simulink model "Elevator_correction"  (R2024b)
settings: Solver=VariableStepAuto  StartTime=0.0  StopTime=SIM.Tmax  MaxStep=SIM.Step_max  RelTol=1e-3
InitFcn:
  | Initialisation
values from neighbouring files (symbols this model uses):
  Kr = 12    [Initialisation.m]
  Mc = 1000.0    (= 1000)    [Initialisation.m]
  Me = 800.0    (= 800)    [Initialisation.m]
  Rp = 0.1    [Initialisation.m]
  Ured = 3.0/pi*sqrt(2.0)*sqrt(3.0)*230.0    [Initialisation.m]
undefined symbols (not defined in the file or in its folder): cycle, IN_filter, MOT, Scap
settings Model: Creator=philippe.barrade  LastModifiedBy=philippe.barrade
settings SolverCC: AlgebraicLoopSolver=TrustRegion
settings DataIOCC: ReturnWorkspaceOutputs=off
settings DebuggingCC: UnconnectedInputMsg=warning  UnconnectedOutputMsg=warning  UnconnectedLineMsg=warning  ArithmeticOperatorsInVariantConditions=warning
settings ModelReferenceCC: EnableRefExpFcnMdlSchedulingChecks=on
settings SFSimCC: SimUseLocalCustomCode=off  CustomCodeUndefinedFunction=UseInterfaceOnly
settings RTWCC: RTWUseLocalCustomCode=off  GPUComputeCapability=3.5
settings CodeAppCC: StateflowObjectComments=on

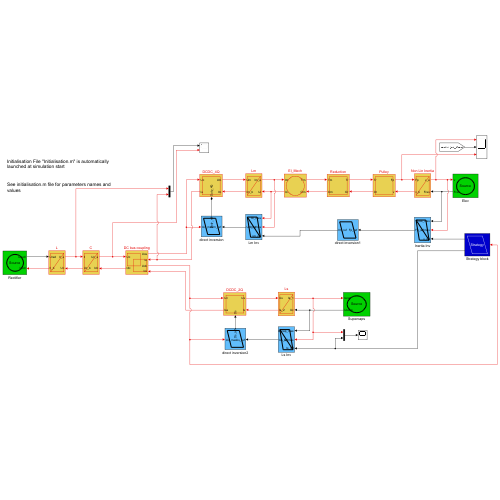
[thumbnail: Simulink's stored preview of the top-level diagram]
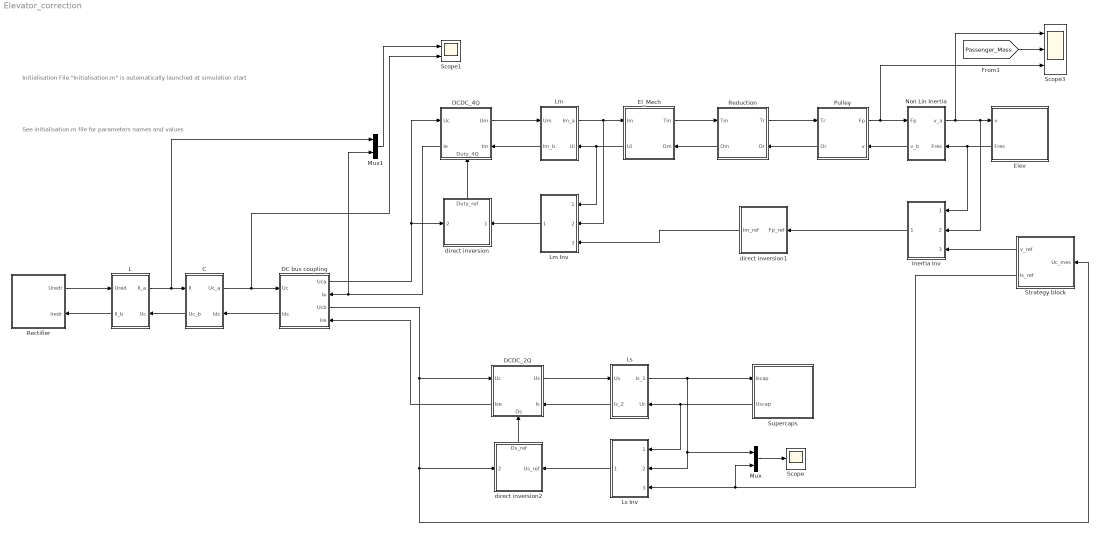
== system Elevator_correction ==
  note: Initialisation File "Initialisation.m" is automatically launched at simulation start
  note: See initialisation.m file for parameters names and values
  C : Subsystem  mask(CM){}
      settings: PortSchema="{\"entries\":[{\"content\":{\"sides\":[{\"content\":{\"connectorIds\":[\"In1\",\"Out2\"]},\"type\":\"ConnectorPlacement.EquallySpacedRectSide\",\"uuid\":\"af5f45e0-9d2b-440a-ad04-5e1193860bd0\"},{\"content\":{\"connectorIds\":[\"Out1\",\"In2\"],\"side\":\"RIGHT\"},\"type\":\"ConnectorPlacement.EquallySpacedRectSide\",\"uuid\":\"8de6af24-0ac6-4b19-a2ba-5daa5911acc7\"},{\"content\":{\"connectorIds\":[],\"side\":\"TOP\"},\"type\":\"ConnectorPlacement.EquallySpacedRectSide\",\"uuid\":\"acb7e0d5-07ac-49d2-a96a-2a7cab5175a2\"}]},\"type\":\"ConnectorPlacement.EquallySpacedConnector\",\"uuid\":\"c84922a6-ff22-4e39-b94d-9f3f8f0085b4\"}],\"packageUris\":[\"http://schema.mathworks.com/mf0/Connector/R2020b\"],\"version\":\"1.0\"}"
      mask Display: plot(0,0,100,100,[10,10,90,90,10],[90,10,10,90,90], [10,90],[10,90])
  DC bus coupling : Subsystem  mask(CM){}
      settings: PortSchema="{\"entries\":[{\"content\":{\"sides\":[{\"content\":{\"connectorIds\":[\"In1\",\"Out3\"]},\"type\":\"ConnectorPlacement.EquallySpacedRectSide\",\"uuid\":\"a0cc6eb3-0f35-4a31-afc0-a3cae9b9d5bb\"},{\"content\":{\"connectorIds\":[\"Out1\",\"In2\",\"Out2\",\"In3\"],\"side\":\"RIGHT\"},\"type\":\"ConnectorPlacement.EquallySpacedRectSide\",\"uuid\":\"f0fc86c1-6f18-402b-9eea-d081ace87e62\"},{\"content\":{\"connectorIds\":[],\"side\":\"TOP\"},\"type\":\"ConnectorPlacement.EquallySpacedRectSide\",\"uuid\":\"dfd8824c-ea43-4486-a7b0-05621e67d875\"}]},\"type\":\"ConnectorPlacement.EquallySpacedConnector\",\"uuid\":\"18c849d2-2a12-4239-b86e-b7a06eec8617\"}],\"packageUris\":[\"http://schema.mathworks.com/mf0/Connector/R2020b\"],\"version\":\"1.0\"}"
      mask Display: plot(0,0,100,100,[35,35,95,95,35],[65,10,10,65,65], [5,5,65,65,5],[90,35,35,90,90])
  DCDC_2Q : Subsystem  mask(Hacheur){}
      settings: PortSchema="{\"entries\":[{\"content\":{\"sides\":[{\"content\":{\"connectorIds\":[\"In1\",\"Out2\"]},\"type\":\"ConnectorPlacement.EquallySpacedRectSide\",\"uuid\":\"18b8dea3-c73c-4489-bf41-881ff948b4bd\"},{\"content\":{\"connectorIds\":[\"Out1\",\"In3\"],\"side\":\"RIGHT\"},\"type\":\"ConnectorPlacement.EquallySpacedRectSide\",\"uuid\":\"3421d2ab-808d-44dd-9f9d-6c595338ccbb\"},{\"content\":{\"connectorIds\":[],\"side\":\"TOP\"},\"type\":\"ConnectorPlacement.EquallySpacedRectSide\",\"uuid\":\"948f89bd-2b52-44e4-9785-94aa615b18dd\"},{\"content\":{\"connectorIds\":[\"In2\"],\"side\":\"BOTTOM\"},\"type\":\"ConnectorPlacement.EquallySpacedRectSide\",\"uuid\":\"f632fc7f-d418-4a7f-b063-8935e3a44c68\"}]},\"type\":\"ConnectorPlacement.EquallySpacedConnector\",\"uuid\":\"698b37cd-a833-4d3c-8172-8b0b4e01ebf3\"}],\"packageUris\":[\"http://schema.mathworks.com/mf0/Connector/R2020b\"],\"version\":\"1.0\"}"
      mask Display: plot(0,0,100,100,[10,10,90,90,10],[90,10,10,90,90])
  DCDC_4Q : Subsystem  mask(Hacheur){}
      settings: PortSchema="{\"entries\":[{\"content\":{\"sides\":[{\"content\":{\"connectorIds\":[\"In1\",\"Out2\"]},\"type\":\"ConnectorPlacement.EquallySpacedRectSide\",\"uuid\":\"18b8dea3-c73c-4489-bf41-881ff948b4bd\"},{\"content\":{\"connectorIds\":[\"Out1\",\"In3\"],\"side\":\"RIGHT\"},\"type\":\"ConnectorPlacement.EquallySpacedRectSide\",\"uuid\":\"3421d2ab-808d-44dd-9f9d-6c595338ccbb\"},{\"content\":{\"connectorIds\":[],\"side\":\"TOP\"},\"type\":\"ConnectorPlacement.EquallySpacedRectSide\",\"uuid\":\"948f89bd-2b52-44e4-9785-94aa615b18dd\"},{\"content\":{\"connectorIds\":[\"In2\"],\"side\":\"BOTTOM\"},\"type\":\"ConnectorPlacement.EquallySpacedRectSide\",\"uuid\":\"2b91a71a-e743-46c5-9fd2-ea2ea7735bb5\"}]},\"type\":\"ConnectorPlacement.EquallySpacedConnector\",\"uuid\":\"698b37cd-a833-4d3c-8172-8b0b4e01ebf3\"}],\"packageUris\":[\"http://schema.mathworks.com/mf0/Connector/R2020b\"],\"version\":\"1.0\"}"
      mask Display: plot(0,0,100,100,[10,10,90,90,10],[90,10,10,90,90])
  El_Mech : Subsystem
      settings: PortSchema="{\"entries\":[{\"content\":{\"sides\":[{\"content\":{\"connectorIds\":[\"In1\",\"Out2\"]},\"type\":\"ConnectorPlacement.EquallySpacedRectSide\",\"uuid\":\"af5f45e0-9d2b-440a-ad04-5e1193860bd0\"},{\"content\":{\"connectorIds\":[\"Out1\",\"In2\"],\"side\":\"RIGHT\"},\"type\":\"ConnectorPlacement.EquallySpacedRectSide\",\"uuid\":\"8de6af24-0ac6-4b19-a2ba-5daa5911acc7\"},{\"content\":{\"connectorIds\":[],\"side\":\"TOP\"},\"type\":\"ConnectorPlacement.EquallySpacedRectSide\",\"uuid\":\"acb7e0d5-07ac-49d2-a96a-2a7cab5175a2\"}]},\"type\":\"ConnectorPlacement.EquallySpacedConnector\",\"uuid\":\"c84922a6-ff22-4e39-b94d-9f3f8f0085b4\"}],\"packageUris\":[\"http://schema.mathworks.com/mf0/Connector/R2020b\"],\"version\":\"1.0\"}"
      mask Display: plot(0,0,100,100, 1.4*[50,57.68,60.77,63.08,64.97,66.58,68,69.26,70.4, 	71.42,72.36,78.28,80,78.28,72.36,71.42,70.4, 	69.26,68,66.58,64.97,63.08,60.77,57.68,50,42.32, 	39.23,36.92,35.03,33.42,32,30.74,29.6,28.58, 	27.64,21.72,20,21.72,27.64,28.58,29.6,30.74,32, 	33.42,35.03,36.92,39.23,42.32,50]-20, 1.4*[20,21,22,23,24,25,26,27,28,29,30,40,50,60,70,71,72, 	73,74,75,76,77,78,79,80,79,78,77,76,75,74,73,72, 	71,70,60,50,40,30,29,28,27,26,25,24,23,22,21,20]-20)
  Elev : Subsystem
      settings: PortSchema="{\"entries\":[{\"content\":{\"sides\":[{\"content\":{\"connectorIds\":[\"In1\",\"Out1\"]},\"type\":\"ConnectorPlacement.EquallySpacedRectSide\",\"uuid\":\"5a8fdec0-a98b-43d7-a4cd-372895ae0c1b\"},{\"content\":{\"connectorIds\":[],\"side\":\"RIGHT\"},\"type\":\"ConnectorPlacement.EquallySpacedRectSide\",\"uuid\":\"94211a24-953d-4ef9-bbc7-a0604a4babfb\"},{\"content\":{\"connectorIds\":[],\"side\":\"TOP\"},\"type\":\"ConnectorPlacement.EquallySpacedRectSide\",\"uuid\":\"df264a2a-7001-4aa8-9401-af00637c2dcd\"}]},\"type\":\"ConnectorPlacement.EquallySpacedConnector\",\"uuid\":\"5b044fdd-039d-40b1-9820-1583afc6fd22\"}],\"packageUris\":[\"http://schema.mathworks.com/mf0/Connector/R2020b\"],\"version\":\"1.0\"}"
      mask Display:
      | plot(0,0,100,100, 1.2*[50,57.68,60.77,63.08,64.97,66.58,68,69.26,70.4, 	71.42,72.36,78.28,80,78.28,72.36,71.42,70.4, 	69.26,68,66.58,64.97,63.08,60.77,57.68,50,42.32, 	39.23,36.92,35.03,33.42,32,30.74,29.6,28.58, 	27.64,21.72,20,21.72,27.64,28.58,29.6,30.74,32, 	33.42,35.03,36.92,39.23,42.32,50]-10, 1.2*[20,21,22,23,24,25,26,27,28,29,30,40,50,60,70,71,72, 	73,74,75,76,77,78,79,80,79,78,77,76,75,74,73,72, 	71,70,60,50,40,30,29,28,27,26,25,24,23,22,21,20]-10)
      | disp('Source')
  Inertia Inv : Subsystem
      mask Display: plot(0,0,100,100, [10,30,90,70,10,90],[90,10,10,90,90,10])
  L : Subsystem  mask(CM){}
      settings: PortSchema="{\"entries\":[{\"content\":{\"sides\":[{\"content\":{\"connectorIds\":[\"In1\",\"Out2\"]},\"type\":\"ConnectorPlacement.EquallySpacedRectSide\",\"uuid\":\"af5f45e0-9d2b-440a-ad04-5e1193860bd0\"},{\"content\":{\"connectorIds\":[\"Out1\",\"In2\"],\"side\":\"RIGHT\"},\"type\":\"ConnectorPlacement.EquallySpacedRectSide\",\"uuid\":\"8de6af24-0ac6-4b19-a2ba-5daa5911acc7\"},{\"content\":{\"connectorIds\":[],\"side\":\"TOP\"},\"type\":\"ConnectorPlacement.EquallySpacedRectSide\",\"uuid\":\"acb7e0d5-07ac-49d2-a96a-2a7cab5175a2\"}]},\"type\":\"ConnectorPlacement.EquallySpacedConnector\",\"uuid\":\"c84922a6-ff22-4e39-b94d-9f3f8f0085b4\"}],\"packageUris\":[\"http://schema.mathworks.com/mf0/Connector/R2020b\"],\"version\":\"1.0\"}"
      mask Display: plot(0,0,100,100,[10,10,90,90,10],[90,10,10,90,90], [10,90],[10,90])
  Lm : Subsystem  mask(CM){}
      settings: PortSchema="{\"entries\":[{\"content\":{\"sides\":[{\"content\":{\"connectorIds\":[\"In1\",\"Out2\"]},\"type\":\"ConnectorPlacement.EquallySpacedRectSide\",\"uuid\":\"af5f45e0-9d2b-440a-ad04-5e1193860bd0\"},{\"content\":{\"connectorIds\":[\"Out1\",\"In2\"],\"side\":\"RIGHT\"},\"type\":\"ConnectorPlacement.EquallySpacedRectSide\",\"uuid\":\"8de6af24-0ac6-4b19-a2ba-5daa5911acc7\"},{\"content\":{\"connectorIds\":[],\"side\":\"TOP\"},\"type\":\"ConnectorPlacement.EquallySpacedRectSide\",\"uuid\":\"acb7e0d5-07ac-49d2-a96a-2a7cab5175a2\"}]},\"type\":\"ConnectorPlacement.EquallySpacedConnector\",\"uuid\":\"c84922a6-ff22-4e39-b94d-9f3f8f0085b4\"}],\"packageUris\":[\"http://schema.mathworks.com/mf0/Connector/R2020b\"],\"version\":\"1.0\"}"
      mask Display: plot(0,0,100,100,[10,10,90,90,10],[90,10,10,90,90], [10,90],[10,90])
  Lm Inv : Subsystem
      mask Display: plot(0,0,100,100, [10,30,90,70,10,90],[90,10,10,90,90,10])
  Ls : Subsystem  mask(CM){}
      settings: PortSchema="{\"entries\":[{\"content\":{\"sides\":[{\"content\":{\"connectorIds\":[\"In1\",\"Out2\"]},\"type\":\"ConnectorPlacement.EquallySpacedRectSide\",\"uuid\":\"af5f45e0-9d2b-440a-ad04-5e1193860bd0\"},{\"content\":{\"connectorIds\":[\"Out1\",\"In2\"],\"side\":\"RIGHT\"},\"type\":\"ConnectorPlacement.EquallySpacedRectSide\",\"uuid\":\"8de6af24-0ac6-4b19-a2ba-5daa5911acc7\"},{\"content\":{\"connectorIds\":[],\"side\":\"TOP\"},\"type\":\"ConnectorPlacement.EquallySpacedRectSide\",\"uuid\":\"acb7e0d5-07ac-49d2-a96a-2a7cab5175a2\"}]},\"type\":\"ConnectorPlacement.EquallySpacedConnector\",\"uuid\":\"c84922a6-ff22-4e39-b94d-9f3f8f0085b4\"}],\"packageUris\":[\"http://schema.mathworks.com/mf0/Connector/R2020b\"],\"version\":\"1.0\"}"
      mask Display: plot(0,0,100,100,[10,10,90,90,10],[90,10,10,90,90], [10,90],[10,90])
  Ls Inv : Subsystem
      mask Display: plot(0,0,100,100, [10,30,90,70,10,90],[90,10,10,90,90,10])
  Mux : Mux  Inputs=2
  Mux1 : Mux  Inputs=2
  Non Lin Inertia : Subsystem  mask(CM){}
      settings: PortSchema="{\"entries\":[{\"content\":{\"sides\":[{\"content\":{\"connectorIds\":[\"In1\",\"Out2\"]},\"type\":\"ConnectorPlacement.EquallySpacedRectSide\",\"uuid\":\"af5f45e0-9d2b-440a-ad04-5e1193860bd0\"},{\"content\":{\"connectorIds\":[\"Out1\",\"In2\"],\"side\":\"RIGHT\"},\"type\":\"ConnectorPlacement.EquallySpacedRectSide\",\"uuid\":\"8de6af24-0ac6-4b19-a2ba-5daa5911acc7\"},{\"content\":{\"connectorIds\":[],\"side\":\"TOP\"},\"type\":\"ConnectorPlacement.EquallySpacedRectSide\",\"uuid\":\"acb7e0d5-07ac-49d2-a96a-2a7cab5175a2\"}]},\"type\":\"ConnectorPlacement.EquallySpacedConnector\",\"uuid\":\"c84922a6-ff22-4e39-b94d-9f3f8f0085b4\"}],\"packageUris\":[\"http://schema.mathworks.com/mf0/Connector/R2020b\"],\"version\":\"1.0\"}"
      mask Display: plot(0,0,100,100,[10,10,90,90,10],[90,10,10,90,90], [10,90],[10,90])
  Pulley : Subsystem  mask(Hacheur){}
      settings: PortSchema="{\"entries\":[{\"content\":{\"sides\":[{\"content\":{\"connectorIds\":[\"In1\",\"Out2\"]},\"type\":\"ConnectorPlacement.EquallySpacedRectSide\",\"uuid\":\"af5f45e0-9d2b-440a-ad04-5e1193860bd0\"},{\"content\":{\"connectorIds\":[\"Out1\",\"In2\"],\"side\":\"RIGHT\"},\"type\":\"ConnectorPlacement.EquallySpacedRectSide\",\"uuid\":\"8de6af24-0ac6-4b19-a2ba-5daa5911acc7\"},{\"content\":{\"connectorIds\":[],\"side\":\"TOP\"},\"type\":\"ConnectorPlacement.EquallySpacedRectSide\",\"uuid\":\"acb7e0d5-07ac-49d2-a96a-2a7cab5175a2\"}]},\"type\":\"ConnectorPlacement.EquallySpacedConnector\",\"uuid\":\"c84922a6-ff22-4e39-b94d-9f3f8f0085b4\"}],\"packageUris\":[\"http://schema.mathworks.com/mf0/Connector/R2020b\"],\"version\":\"1.0\"}"
      mask Display: plot(0,0,100,100,[10,10,90,90,10],[90,10,10,90,90])
  Rectifier : Subsystem
      settings: PortSchema="{\"entries\":[{\"content\":{\"sides\":[{\"content\":{\"connectorIds\":[]},\"type\":\"ConnectorPlacement.EquallySpacedRectSide\",\"uuid\":\"5a8fdec0-a98b-43d7-a4cd-372895ae0c1b\"},{\"content\":{\"connectorIds\":[\"Out1\",\"In1\"],\"side\":\"RIGHT\"},\"type\":\"ConnectorPlacement.EquallySpacedRectSide\",\"uuid\":\"94211a24-953d-4ef9-bbc7-a0604a4babfb\"},{\"content\":{\"connectorIds\":[],\"side\":\"TOP\"},\"type\":\"ConnectorPlacement.EquallySpacedRectSide\",\"uuid\":\"df264a2a-7001-4aa8-9401-af00637c2dcd\"}]},\"type\":\"ConnectorPlacement.EquallySpacedConnector\",\"uuid\":\"5b044fdd-039d-40b1-9820-1583afc6fd22\"}],\"packageUris\":[\"http://schema.mathworks.com/mf0/Connector/R2020b\"],\"version\":\"1.0\"}"
      mask Display:
      | plot(0,0,100,100, 1.2*[50,57.68,60.77,63.08,64.97,66.58,68,69.26,70.4, 	71.42,72.36,78.28,80,78.28,72.36,71.42,70.4, 	69.26,68,66.58,64.97,63.08,60.77,57.68,50,42.32, 	39.23,36.92,35.03,33.42,32,30.74,29.6,28.58, 	27.64,21.72,20,21.72,27.64,28.58,29.6,30.74,32, 	33.42,35.03,36.92,39.23,42.32,50]-10, 1.2*[20,21,22,23,24,25,26,27,28,29,30,40,50,60,70,71,72, 	73,74,75,76,77,78,79,80,79,78,77,76,75,74,73,72, 	71,70,60,50,40,30,29,28,27,26,25,24,23,22,21,20]-10)
      | disp('Source')
  Reduction : Subsystem  mask(Hacheur){}
      settings: PortSchema="{\"entries\":[{\"content\":{\"sides\":[{\"content\":{\"connectorIds\":[\"In1\",\"Out2\"]},\"type\":\"ConnectorPlacement.EquallySpacedRectSide\",\"uuid\":\"af5f45e0-9d2b-440a-ad04-5e1193860bd0\"},{\"content\":{\"connectorIds\":[\"Out1\",\"In2\"],\"side\":\"RIGHT\"},\"type\":\"ConnectorPlacement.EquallySpacedRectSide\",\"uuid\":\"8de6af24-0ac6-4b19-a2ba-5daa5911acc7\"},{\"content\":{\"connectorIds\":[],\"side\":\"TOP\"},\"type\":\"ConnectorPlacement.EquallySpacedRectSide\",\"uuid\":\"acb7e0d5-07ac-49d2-a96a-2a7cab5175a2\"}]},\"type\":\"ConnectorPlacement.EquallySpacedConnector\",\"uuid\":\"c84922a6-ff22-4e39-b94d-9f3f8f0085b4\"}],\"packageUris\":[\"http://schema.mathworks.com/mf0/Connector/R2020b\"],\"version\":\"1.0\"}"
      mask Display: plot(0,0,100,100,[10,10,90,90,10],[90,10,10,90,90])
  Scope : Scope
  Scope1 : Scope  NumInputPorts=2
  Scope3 : Scope  NumInputPorts=3
  Strategy block : Subsystem
      mask Display:
      | color('white')
      | plot(0,0,100,100,[10,30,90,70,10],[90,10,10,90,90])
      | disp('Strategy')
  Supercaps : Subsystem
      settings: PortSchema="{\"entries\":[{\"content\":{\"sides\":[{\"content\":{\"connectorIds\":[\"In1\",\"Out1\"]},\"type\":\"ConnectorPlacement.EquallySpacedRectSide\",\"uuid\":\"5a8fdec0-a98b-43d7-a4cd-372895ae0c1b\"},{\"content\":{\"connectorIds\":[],\"side\":\"RIGHT\"},\"type\":\"ConnectorPlacement.EquallySpacedRectSide\",\"uuid\":\"94211a24-953d-4ef9-bbc7-a0604a4babfb\"},{\"content\":{\"connectorIds\":[],\"side\":\"TOP\"},\"type\":\"ConnectorPlacement.EquallySpacedRectSide\",\"uuid\":\"df264a2a-7001-4aa8-9401-af00637c2dcd\"}]},\"type\":\"ConnectorPlacement.EquallySpacedConnector\",\"uuid\":\"5b044fdd-039d-40b1-9820-1583afc6fd22\"}],\"packageUris\":[\"http://schema.mathworks.com/mf0/Connector/R2020b\"],\"version\":\"1.0\"}"
      mask Display:
      | plot(0,0,100,100, 1.2*[50,57.68,60.77,63.08,64.97,66.58,68,69.26,70.4, 	71.42,72.36,78.28,80,78.28,72.36,71.42,70.4, 	69.26,68,66.58,64.97,63.08,60.77,57.68,50,42.32, 	39.23,36.92,35.03,33.42,32,30.74,29.6,28.58, 	27.64,21.72,20,21.72,27.64,28.58,29.6,30.74,32, 	33.42,35.03,36.92,39.23,42.32,50]-10, 1.2*[20,21,22,23,24,25,26,27,28,29,30,40,50,60,70,71,72, 	73,74,75,76,77,78,79,80,79,78,77,76,75,74,73,72, 	71,70,60,50,40,30,29,28,27,26,25,24,23,22,21,20]-10)
      | disp('Source')
  direct inversion : Subsystem
      settings: PortSchema="{\"entries\":[{\"content\":{\"sides\":[{\"content\":{\"connectorIds\":[\"In1\"]},\"type\":\"ConnectorPlacement.EquallySpacedRectSide\",\"uuid\":\"8737cb71-7821-4d4d-8489-35b4051bd236\"},{\"content\":{\"connectorIds\":[\"In2\"],\"side\":\"RIGHT\"},\"type\":\"ConnectorPlacement.EquallySpacedRectSide\",\"uuid\":\"1ea57527-9b6b-4299-8c88-4309fd975928\"},{\"content\":{\"connectorIds\":[\"Out1\"],\"side\":\"TOP\"},\"type\":\"ConnectorPlacement.EquallySpacedRectSide\",\"uuid\":\"ebf1b75b-1a11-404d-8ffd-64faf59355e3\"}]},\"type\":\"ConnectorPlacement.EquallySpacedConnector\",\"uuid\":\"c4d00950-85db-4ba2-a578-5e7ddc75704e\"}],\"packageUris\":[\"http://schema.mathworks.com/mf0/Connector/R2020b\"],\"version\":\"1.0\"}"
      mask Display: plot(0,0,100,100,[10,30,90,70,10],[90,10,10,90,90])
  direct inversion1 : Subsystem
      mask Display: plot(0,0,100,100,[10,30,90,70,10],[90,10,10,90,90])
  direct inversion2 : Subsystem
      settings: PortSchema="{\"entries\":[{\"content\":{\"sides\":[{\"content\":{\"connectorIds\":[\"In1\"]},\"type\":\"ConnectorPlacement.EquallySpacedRectSide\",\"uuid\":\"8737cb71-7821-4d4d-8489-35b4051bd236\"},{\"content\":{\"connectorIds\":[\"In2\"],\"side\":\"RIGHT\"},\"type\":\"ConnectorPlacement.EquallySpacedRectSide\",\"uuid\":\"1ea57527-9b6b-4299-8c88-4309fd975928\"},{\"content\":{\"connectorIds\":[\"Out1\"],\"side\":\"TOP\"},\"type\":\"ConnectorPlacement.EquallySpacedRectSide\",\"uuid\":\"ebf1b75b-1a11-404d-8ffd-64faf59355e3\"}]},\"type\":\"ConnectorPlacement.EquallySpacedConnector\",\"uuid\":\"c4d00950-85db-4ba2-a578-5e7ddc75704e\"}],\"packageUris\":[\"http://schema.mathworks.com/mf0/Connector/R2020b\"],\"version\":\"1.0\"}"
      mask Display: plot(0,0,100,100,[10,30,90,70,10],[90,10,10,90,90])
  wires:
  Rectifier/1(Uredr) -> L/1(Ured)
  L/1(Il_a) -> Mux1/1, C/1(Il)
  C/2(Uc_b) -> L/2(Uc)
  L/2(Il_b) -> Rectifier/1(Iredr)
  DCDC_4Q/1(Um) -> Lm/1(Um)
  Lm/1(Im_a) -> Lm Inv/2(Im_mes), El_Mech/1(Im)
  El_Mech/2(Ui) -> Lm Inv/1(Ui_mes), Lm/2(Ui)
  Lm/2(Im_b) -> DCDC_4Q/3(Im)
  El_Mech/1(Tm) -> Reduction/1(Tm)
  Reduction/2(Om) -> El_Mech/2(Om)
  Pulley/2(Or) -> Reduction/2(Or)
  Reduction/1(Tr) -> Pulley/1(Tr)
  Non Lin Inertia/2(v_b) -> Pulley/2(v)
  Non Lin Inertia/1(v_a) -> Inertia Inv/2(v_mes), Elev/1(v), Scope3/1
  Elev/1(Fres) -> Inertia Inv/1(Fres_mes), Non Lin Inertia/2(Fres)
  Lm Inv/1(Um_ref) -> direct inversion/1(Um_ref)
  Mux/1 -> Scope/1
  direct inversion1/1(Im_ref) -> Lm Inv/3(Im_ref)
  Inertia Inv/1(Fp_ref) -> direct inversion1/1(Fp_ref)
  C/1(Uc_a) -> Scope1/2, DC bus coupling/1(Uc)
  DC bus coupling/3(Idc) -> C/2(Idc)
  DC bus coupling/1(Uca) -> direct inversion/2(Uc_mes), DCDC_4Q/1(Uc)
  DCDC_4Q/2(Ie) -> Mux1/2, DC bus coupling/2(Ie)
  DC bus coupling/2(Ucb) -> direct inversion2/2(Uc_mes), Strategy block/1(Uc_mes), DCDC_2Q/1(Uc)
  DCDC_2Q/2(Ise) -> DC bus coupling/3(Ire)
  direct inversion2/1(Ds_ref) -> DCDC_2Q/2(Ds)
  Strategy block/1(v_ref) -> Inertia Inv/3(v_ref)
  DCDC_2Q/1(Us) -> Ls/1(Us)
  Ls/1(Is_1) -> Mux/1, Ls Inv/2(Is_mes), Supercaps/1(Iscap)
  Supercaps/1(Uscap) -> Ls Inv/1(Uscap_mes), Ls/2(Uc)
  Ls/2(Is_2) -> DCDC_2Q/3(Is)
  Ls Inv/1(Us_ref) -> direct inversion2/1(Us_ref)
  [Passenger_Mass] -> Scope3/2
  Pulley/1(Fp) -> Scope3/3, Non Lin Inertia/1(Fp)
  direct inversion/1(Duty_ref) -> DCDC_4Q/2(Duty_4Q)
  Mux1/1 -> Scope1/1
  Strategy block/2(Is_ref) -> Mux/2, Ls Inv/3(Is_ref)

== system Elevator_correction/C ==
  Il : Inport
  Idc : Inport  Port=2
  Add : Sum  Inputs=+-
  Gain : Gain  Gain=1/IN_filter.C
  Integrator : Integrator  InitialCondition=Ured
  Uc_a : Outport  InitialOutput=0  VectorParamsAs1DForOutWhenUnconnected=off
  Uc_b : Outport  Port=2  InitialOutput=0  VectorParamsAs1DForOutWhenUnconnected=off
  wires:
  Add/1 -> Gain/1
  Gain/1 -> Integrator/1
  Integrator/1 -> Uc_a/1, Uc_b/1
  Il/1 -> Add/1
  Idc/1 -> Add/2

== system Elevator_correction/DC bus coupling ==
  Uc : Inport
  Ie : Inport  Port=2
  Ire : Inport  Port=3
  Add : Sum
  Uca : Outport  InitialOutput=0  VectorParamsAs1DForOutWhenUnconnected=off
  Ucb : Outport  Port=2  InitialOutput=0  VectorParamsAs1DForOutWhenUnconnected=off
  Idc : Outport  Port=3  InitialOutput=0  VectorParamsAs1DForOutWhenUnconnected=off
  wires:
  Uc/1 -> Ucb/1, Uca/1
  Ie/1 -> Add/1
  Ire/1 -> Add/2
  Add/1 -> Idc/1

== system Elevator_correction/DCDC_2Q ==
  Uc : Inport
  Ds : Inport  Port=2
  Is : Inport  Port=3
  Product : Product
  Product1 : Product
  Us : Outport  InitialOutput=0  VectorParamsAs1DForOutWhenUnconnected=off
  Ise : Outport  Port=2  InitialOutput=0  VectorParamsAs1DForOutWhenUnconnected=off
  wires:
  Ds/1 -> Product1/1, Product/2
  Product/1 -> Us/1
  Product1/1 -> Ise/1
  Uc/1 -> Product/1
  Is/1 -> Product1/2

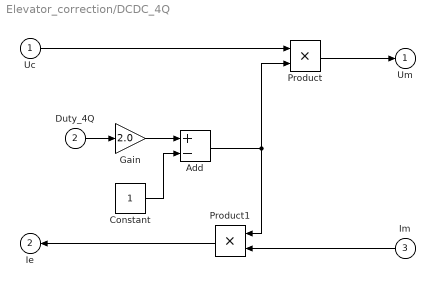
== system Elevator_correction/DCDC_4Q ==
  Uc : Inport
  Duty_4Q : Inport  Port=2
  Im : Inport  Port=3
  Add : Sum  Inputs=+-
  Constant : Constant
  Gain : Gain  Gain=2.0
  Product : Product
  Product1 : Product
  Um : Outport  InitialOutput=0  VectorParamsAs1DForOutWhenUnconnected=off
  Ie : Outport  Port=2  InitialOutput=0  VectorParamsAs1DForOutWhenUnconnected=off
  wires:
  Duty_4Q/1 -> Gain/1
  Product/1 -> Um/1
  Im/1 -> Product1/2
  Product1/1 -> Ie/1
  Gain/1 -> Add/1
  Constant/1 -> Add/2
  Add/1 -> Product1/1, Product/2
  Uc/1 -> Product/1

== system Elevator_correction/El_Mech ==
  Im : Inport
  Om : Inport  Port=2
  Gain : Gain  Gain=MOT.Km
  Gain1 : Gain  Gain=MOT.Km
  Tm : Outport  InitialOutput=0  VectorParamsAs1DForOutWhenUnconnected=off
  Ui : Outport  Port=2  InitialOutput=0  VectorParamsAs1DForOutWhenUnconnected=off
  wires:
  Gain/1 -> Tm/1
  Im/1 -> Gain/1
  Om/1 -> Gain1/1
  Gain1/1 -> Ui/1

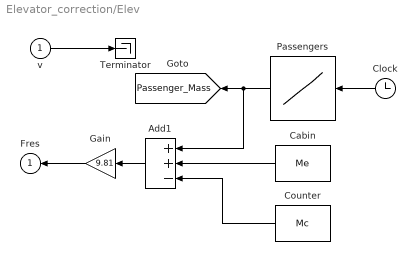
== system Elevator_correction/Elev ==
  v : Inport
  Add1 : Sum  Inputs=++-
  Cabin : Constant  Value=Me
  Clock : Clock
  Counter : Constant  Value=Mc
  Gain : Gain  Gain=9.81
  Passengers : Lookup_n-D  NumberOfTableDimensions=1  BreakpointsForDimension1=cycle.time_ref  Table=cycle.mass_ref  InternalRulePriority=Speed  RndMeth=Simplest
  Terminator : Terminator
  Fres : Outport  InitialOutput=0  VectorParamsAs1DForOutWhenUnconnected=off
  tag scope: Passenger_Mass=global
  wires:
  Add1/1 -> Gain/1
  v/1 -> Terminator/1
  Clock/1 -> Passengers/1
  Passengers/1 -> [Passenger_Mass], Add1/1
  Cabin/1 -> Add1/2
  Counter/1 -> Add1/3
  Gain/1 -> Fres/1

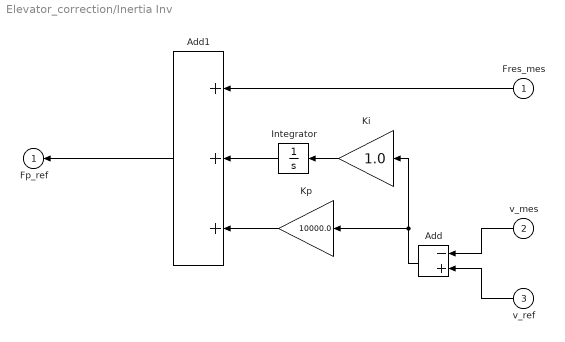
== system Elevator_correction/Inertia Inv ==
  Fres_mes : Inport
  v_mes : Inport  Port=2
  v_ref : Inport  Port=3
  Add : Sum  Inputs=-+
  Add1 : Sum  Inputs=+++
  Integrator : Integrator
  Ki : Gain  Gain=1.0
  Kp : Gain  Gain=10000.0
  Fp_ref : Outport  InitialOutput=0  VectorParamsAs1DForOutWhenUnconnected=off
  wires:
  v_ref/1 -> Add/2
  v_mes/1 -> Add/1
  Add/1 -> Ki/1, Kp/1
  Integrator/1 -> Add1/2
  Kp/1 -> Add1/3
  Ki/1 -> Integrator/1
  Fres_mes/1 -> Add1/1
  Add1/1 -> Fp_ref/1

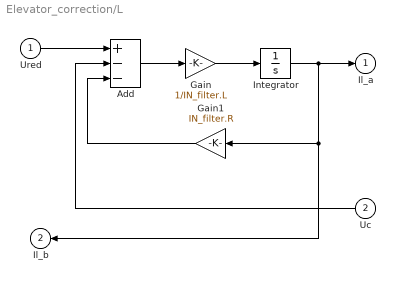
== system Elevator_correction/L ==
  Ured : Inport
  Uc : Inport  Port=2
  Add : Sum  Inputs=+--
  Gain : Gain  Gain=1/IN_filter.L
  Gain1 : Gain  Gain=IN_filter.R
  Integrator : Integrator  LowerSaturationLimit=0.0
  Il_a : Outport  InitialOutput=0  VectorParamsAs1DForOutWhenUnconnected=off
  Il_b : Outport  Port=2  InitialOutput=0  VectorParamsAs1DForOutWhenUnconnected=off
  wires:
  Add/1 -> Gain/1
  Gain/1 -> Integrator/1
  Integrator/1 -> Il_b/1, Gain1/1, Il_a/1
  Ured/1 -> Add/1
  Uc/1 -> Add/2
  Gain1/1 -> Add/3

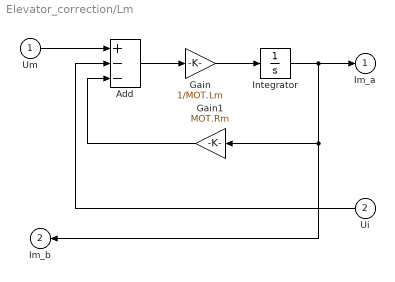
== system Elevator_correction/Lm ==
  Um : Inport
  Ui : Inport  Port=2
  Add : Sum  Inputs=+--
  Gain : Gain  Gain=1/MOT.Lm
  Gain1 : Gain  Gain=MOT.Rm
  Integrator : Integrator
  Im_a : Outport  InitialOutput=0  VectorParamsAs1DForOutWhenUnconnected=off
  Im_b : Outport  Port=2  InitialOutput=0  VectorParamsAs1DForOutWhenUnconnected=off
  wires:
  Add/1 -> Gain/1
  Gain/1 -> Integrator/1
  Integrator/1 -> Im_b/1, Gain1/1, Im_a/1
  Um/1 -> Add/1
  Ui/1 -> Add/2
  Gain1/1 -> Add/3

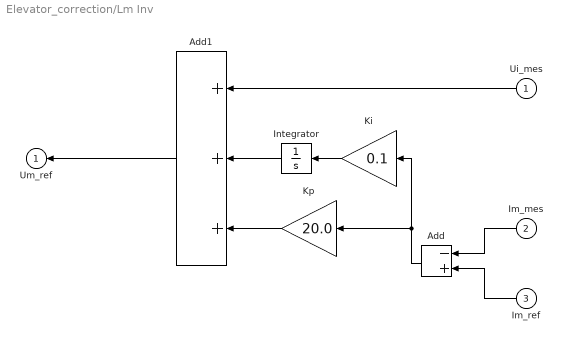
== system Elevator_correction/Lm Inv ==
  Ui_mes : Inport
  Im_mes : Inport  Port=2
  Im_ref : Inport  Port=3
  Add : Sum  Inputs=-+
  Add1 : Sum  Inputs=+++
  Integrator : Integrator
  Ki : Gain  Gain=0.1
  Kp : Gain  Gain=20.0
  Um_ref : Outport  InitialOutput=0  VectorParamsAs1DForOutWhenUnconnected=off
  wires:
  Im_ref/1 -> Add/2
  Im_mes/1 -> Add/1
  Add/1 -> Ki/1, Kp/1
  Integrator/1 -> Add1/2
  Kp/1 -> Add1/3
  Ki/1 -> Integrator/1
  Ui_mes/1 -> Add1/1
  Add1/1 -> Um_ref/1

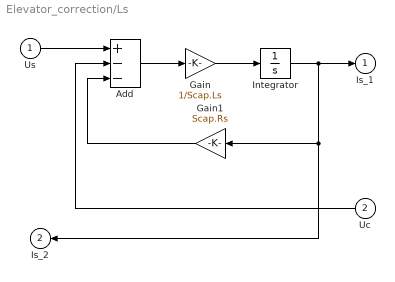
== system Elevator_correction/Ls ==
  Us : Inport
  Uc : Inport  Port=2
  Add : Sum  Inputs=+--
  Gain : Gain  Gain=1/Scap.Ls
  Gain1 : Gain  Gain=Scap.Rs
  Integrator : Integrator  LowerSaturationLimit=0.0
  Is_1 : Outport  InitialOutput=0  VectorParamsAs1DForOutWhenUnconnected=off
  Is_2 : Outport  Port=2  InitialOutput=0  VectorParamsAs1DForOutWhenUnconnected=off
  wires:
  Add/1 -> Gain/1
  Gain/1 -> Integrator/1
  Integrator/1 -> Is_2/1, Gain1/1, Is_1/1
  Us/1 -> Add/1
  Uc/1 -> Add/2
  Gain1/1 -> Add/3

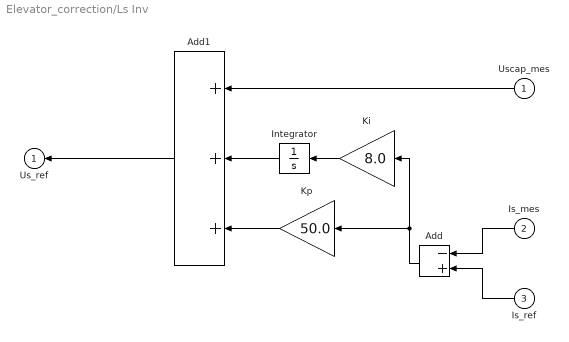
== system Elevator_correction/Ls Inv ==
  Uscap_mes : Inport
  Is_mes : Inport  Port=2
  Is_ref : Inport  Port=3
  Add : Sum  Inputs=-+
  Add1 : Sum  Inputs=+++
  Integrator : Integrator
  Ki : Gain  Gain=8.0
  Kp : Gain  Gain=50.0
  Us_ref : Outport  InitialOutput=0  VectorParamsAs1DForOutWhenUnconnected=off
  wires:
  Is_ref/1 -> Add/2
  Is_mes/1 -> Add/1
  Add/1 -> Ki/1, Kp/1
  Integrator/1 -> Add1/2
  Kp/1 -> Add1/3
  Ki/1 -> Integrator/1
  Uscap_mes/1 -> Add1/1
  Add1/1 -> Us_ref/1

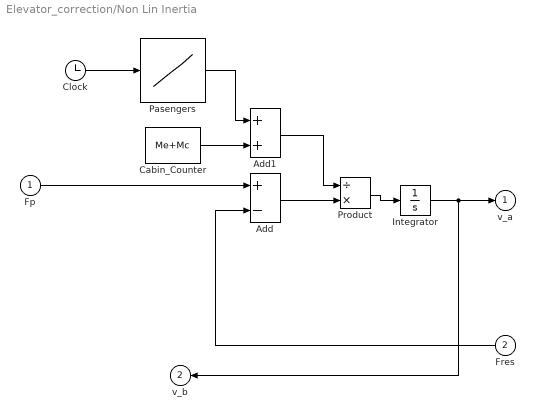
== system Elevator_correction/Non Lin Inertia ==
  Fp : Inport
  Fres : Inport  Port=2
  Add : Sum  Inputs=+-
  Add1 : Sum
  Cabin_Counter : Constant  Value=Me+Mc
  Clock : Clock
  Integrator : Integrator
  Pasengers : Lookup_n-D  NumberOfTableDimensions=1  BreakpointsForDimension1=cycle.time_ref  Table=cycle.mass_ref  InternalRulePriority=Speed  RndMeth=Simplest
  Product : Product  Inputs=/*
  v_a : Outport  InitialOutput=0  VectorParamsAs1DForOutWhenUnconnected=off
  v_b : Outport  Port=2  InitialOutput=0  VectorParamsAs1DForOutWhenUnconnected=off
  wires:
  Integrator/1 -> v_b/1, v_a/1
  Fp/1 -> Add/1
  Fres/1 -> Add/2
  Clock/1 -> Pasengers/1
  Pasengers/1 -> Add1/1
  Cabin_Counter/1 -> Add1/2
  Product/1 -> Integrator/1
  Add/1 -> Product/2
  Add1/1 -> Product/1

== system Elevator_correction/Pulley ==
  Tr : Inport
  v : Inport  Port=2
  Gain : Gain  Gain=1/Rp
  Gain1 : Gain  Gain=1/Rp
  Fp : Outport  InitialOutput=0  VectorParamsAs1DForOutWhenUnconnected=off
  Or : Outport  Port=2  InitialOutput=0  VectorParamsAs1DForOutWhenUnconnected=off
  wires:
  v/1 -> Gain1/1
  Tr/1 -> Gain/1
  Gain/1 -> Fp/1
  Gain1/1 -> Or/1

== system Elevator_correction/Rectifier ==
  Iredr : Inport
  Gain : Gain  Gain=-1/0.0001
  Integrator : Integrator  InitialCondition=Ured  LimitOutput=on  LowerSaturationLimit=Ured
  Uredr : Outport  InitialOutput=0  VectorParamsAs1DForOutWhenUnconnected=off
  wires:
  Iredr/1 -> Gain/1
  Gain/1 -> Integrator/1
  Integrator/1 -> Uredr/1

== system Elevator_correction/Reduction ==
  Tm : Inport
  Or : Inport  Port=2
  Gain : Gain  Gain=Kr
  Gain1 : Gain  Gain=Kr
  Tr : Outport  InitialOutput=0  VectorParamsAs1DForOutWhenUnconnected=off
  Om : Outport  Port=2  InitialOutput=0  VectorParamsAs1DForOutWhenUnconnected=off
  wires:
  Or/1 -> Gain1/1
  Tm/1 -> Gain/1
  Gain/1 -> Tr/1
  Gain1/1 -> Om/1

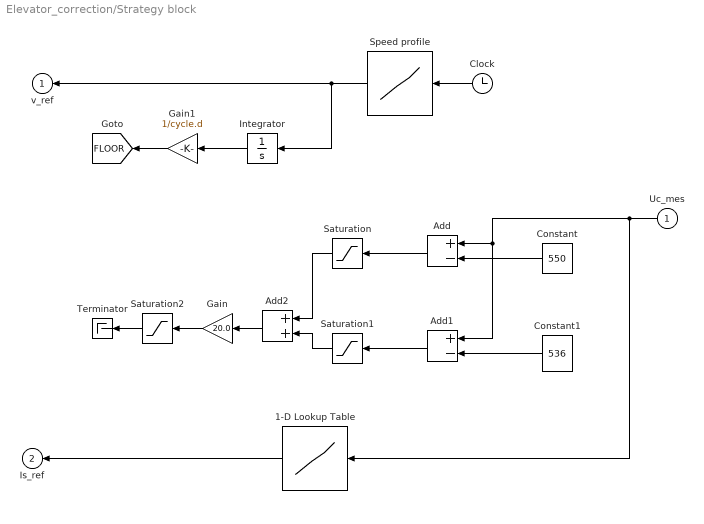
== system Elevator_correction/Strategy block ==
  Uc_mes : Inport
  1-D Lookup Table : Lookup_n-D  NumberOfTableDimensions=1  BreakpointsForDimension1=[536 540 550 560]  Table=[-10 0 5 10]  InternalRulePriority=Speed  RndMeth=Simplest
  Add : Sum  Inputs=+-
  Add1 : Sum  Inputs=+-
  Add2 : Sum
  Clock : Clock
  Constant : Constant  Value=550
  Constant1 : Constant  Value=536
  Gain : Gain  Gain=20.0
  Gain1 : Gain  Gain=1/cycle.d
  Integrator : Integrator
  Saturation : Saturate  UpperLimit=540.0  LowerLimit=0.0
  Saturation1 : Saturate  UpperLimit=0.0  LowerLimit=-200.0
  Saturation2 : Saturate  UpperLimit=10.0  LowerLimit=-10.0
  Speed profile : Lookup_n-D  NumberOfTableDimensions=1  BreakpointsForDimension1=cycle.time_ref  Table=cycle.speed_ref  InternalRulePriority=Speed  RndMeth=Simplest
  Terminator : Terminator
  v_ref : Outport  InitialOutput=0  VectorParamsAs1DForOutWhenUnconnected=off
  Is_ref : Outport  Port=2  InitialOutput=0  VectorParamsAs1DForOutWhenUnconnected=off
  tag scope: FLOOR=global
  wires:
  Clock/1 -> Speed profile/1
  Speed profile/1 -> Integrator/1, v_ref/1
  Constant/1 -> Add/2
  Add/1 -> Saturation/1
  Gain/1 -> Saturation2/1
  Uc_mes/1 -> 1-D Lookup Table/1, Add1/1, Add/1
  Add2/1 -> Gain/1
  Saturation/1 -> Add2/1
  Add1/1 -> Saturation1/1
  Constant1/1 -> Add1/2
  Saturation1/1 -> Add2/2
  Integrator/1 -> Gain1/1
  Gain1/1 -> [FLOOR]
  Saturation2/1 -> Terminator/1
  1-D Lookup Table/1 -> Is_ref/1

== system Elevator_correction/Supercaps ==
  Iscap : Inport
  Constant : Constant  Value=Scap.Uscap
  Terminator : Terminator
  Uscap : Outport  InitialOutput=0  VectorParamsAs1DForOutWhenUnconnected=off
  wires:
  Constant/1 -> Uscap/1
  Iscap/1 -> Terminator/1

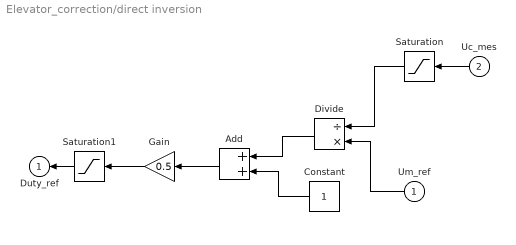
== system Elevator_correction/direct inversion ==
  Um_ref : Inport
  Uc_mes : Inport  Port=2
  Add : Sum
  Constant : Constant
  Divide : Product  Inputs=/*
  Gain : Gain  Gain=0.5
  Saturation : Saturate  UpperLimit=Inf  LowerLimit=1.0
  Saturation1 : Saturate  UpperLimit=1  LowerLimit=0
  Duty_ref : Outport  InitialOutput=0  VectorParamsAs1DForOutWhenUnconnected=off
  wires:
  Uc_mes/1 -> Saturation/1
  Saturation/1 -> Divide/1
  Um_ref/1 -> Divide/2
  Divide/1 -> Add/1
  Constant/1 -> Add/2
  Add/1 -> Gain/1
  Gain/1 -> Saturation1/1
  Saturation1/1 -> Duty_ref/1

== system Elevator_correction/direct inversion1 ==
  Fp_ref : Inport
  Gain : Gain  Gain=1/MOT.Km
  Gain1 : Gain  Gain=1/Kr
  Gain2 : Gain  Gain=Rp
  Im_ref : Outport  InitialOutput=0  VectorParamsAs1DForOutWhenUnconnected=off
  wires:
  Gain/1 -> Im_ref/1
  Gain1/1 -> Gain/1
  Gain2/1 -> Gain1/1
  Fp_ref/1 -> Gain2/1

== system Elevator_correction/direct inversion2 ==
  Us_ref : Inport
  Uc_mes : Inport  Port=2
  Divide : Product  Inputs=/*
  Saturation : Saturate  UpperLimit=Inf  LowerLimit=1.0
  Saturation3 : Saturate  UpperLimit=1  LowerLimit=0
  Ds_ref : Outport  InitialOutput=0  VectorParamsAs1DForOutWhenUnconnected=off
  wires:
  Saturation3/1 -> Ds_ref/1
  Divide/1 -> Saturation3/1
  Uc_mes/1 -> Saturation/1
  Us_ref/1 -> Divide/2
  Saturation/1 -> Divide/1
